simulink model "index_example"  (Simulink 7.0)
settings: Solver=ode23tb  StartTime=0.0  StopTime=50  RelTol=1e-3
libraries: simulink_extras x1
settings Model: Creator=fo1521  LastModifiedBy=fo1521
settings DebuggingCC: SolverPrmCheckMsg=none  MultiTaskDSMMsg=warning  MultiTaskCondExecSysMsg=none  StrictBusMsg=None
settings HardwareCC: TargetHWDeviceType=32-bit Generic
settings RTWCC: IncludeERTFirstTime=on
settings GRTTargetCC: TargetFcnLib=ansi_tfl_tmw.mat

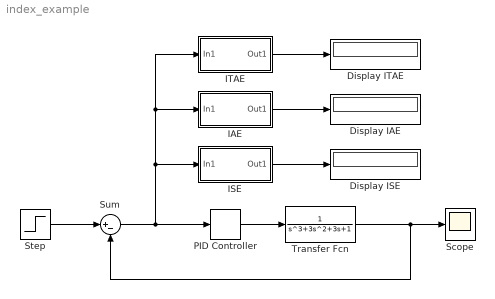
== system index_example ==
  Display IAE : Display
  Display ISE : Display
  Display ITAE : Display
  IAE : Subsystem
      mask Description:
      | IAE performacne index
      | 
      | output = int |input| dt
      mask Display:
      | disp('IAE')
      | port_label('input',1,'e')
      | port_label('output',1,'iae')
  ISE : Subsystem
      mask Description:
      | ISE performance index
      | 
      | output = int (input)^2 dt
      mask Display:
      | disp('ISE')
      | port_label('input',1,'e')
      | port_label('output',1,'ise')
  ITAE : Subsystem
      mask Description:
      | ITAE performance index
      | 
      | output = int t|input| dt
      mask Display:
      | disp('ITAE')
      | port_label('input',1,'e')
      | port_label('output',1,'itae')
  PID Controller : simulink_extras/Additional Linear/PID Controller  SystemSampleTime=-1  P=2  I=1  D=0
  Scope : Scope
  Step : Step  SampleTime=0
  Sum : Sum  Inputs=|+-  OutDataType=sfix(16)  OutScaling=2^0
  Transfer Fcn : TransferFcn  Denominator=[1 3 3 1]
  wires:
  PID Controller/1 -> Transfer Fcn/1
  Sum/1 -> PID Controller/1, ISE/1(In1), IAE/1(In1), ITAE/1(In1)
  Step/1 -> Sum/1
  IAE/1(Out1) -> Display IAE/1
  Transfer Fcn/1 -> Scope/1, Sum/2
  ISE/1(Out1) -> Display ISE/1
  ITAE/1(Out1) -> Display ITAE/1

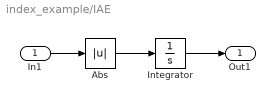
== system index_example/IAE ==
  In1 : Inport
  Abs : Abs
  Integrator : Integrator
  Out1 : Outport
  wires:
  In1/1 -> Abs/1
  Integrator/1 -> Out1/1
  Abs/1 -> Integrator/1

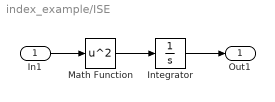
== system index_example/ISE ==
  In1 : Inport
  Integrator : Integrator
  Math Function : Math  Operator=square  OutDataType=sfix(16)  OutScaling=2^0  SaturateOnIntegerOverflow=on
  Out1 : Outport
  wires:
  Math Function/1 -> Integrator/1
  Integrator/1 -> Out1/1
  In1/1 -> Math Function/1

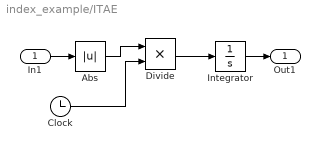
== system index_example/ITAE ==
  In1 : Inport
  Abs : Abs
  Clock : Clock
      settings: Decimation=10
  Divide : Product  Inputs=**  OutDataType=sfix(16)  OutScaling=2^-10
  Integrator : Integrator
  Out1 : Outport
  wires:
  Integrator/1 -> Out1/1
  In1/1 -> Abs/1
  Divide/1 -> Integrator/1
  Abs/1 -> Divide/1
  Clock/1 -> Divide/2
